simulink model "truck_fra_oven_konstant_hastighet"  (R2019b)
settings: Solver=VariableStepAuto  StartTime=0.0  StopTime=10.0  MaxStep=0.01  RelTol=1e-3
settings Model: EnablePacing=on  Creator=hansae  LastModifiedBy=hansae
settings DebuggingCC: UnconnectedInputMsg=none  UnconnectedOutputMsg=none  UnconnectedLineMsg=none  SFMachineParentedDataDiag=error
settings ModelReferenceCC: EnableRefExpFcnMdlSchedulingChecks=off
settings RTWCC: Description=Generic Real-Time Target

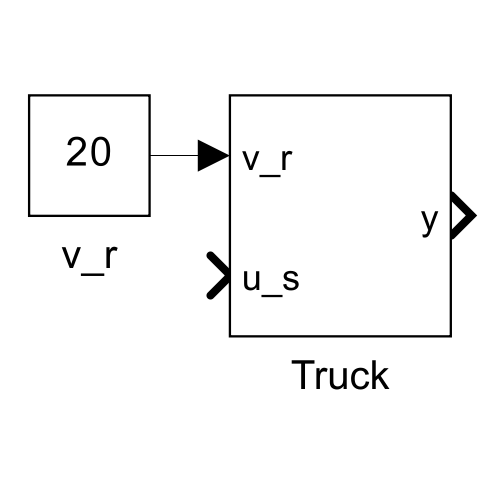
[thumbnail: Simulink's stored preview of the top-level diagram]
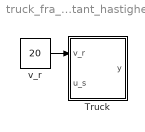
== system truck_fra_oven_konstant_hastighet ==
  Truck : Subsystem
  v_r : Constant  Value=20
  wires:
  v_r/1 -> Truck/1(v_r)

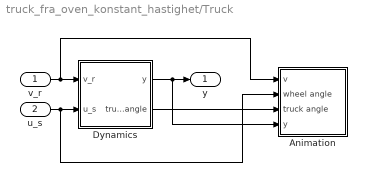
== system truck_fra_oven_konstant_hastighet/Truck ==
  v_r : Inport
  u_s : Inport  Port=2
  Animation : Subsystem
  Dynamics : Subsystem  ClipboardFcn=parameters_truck.m
  y : Outport
  wires:
  Dynamics/1(y) -> Animation/4(y), y/1
  u_s/1 -> Animation/2(wheel angle), Dynamics/2(u_s)
  v_r/1 -> Animation/1(v), Dynamics/1(v_r)
  Dynamics/2(truck angle) -> Animation/3(truck angle)

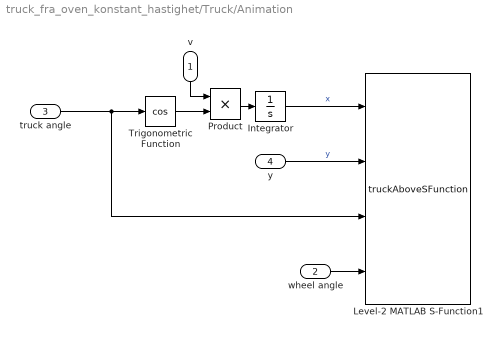
== system truck_fra_oven_konstant_hastighet/Truck/Animation ==
  v : Inport
  wheel angle : Inport  Port=2
  truck angle : Inport  Port=3
  y : Inport  Port=4
  Integrator : Integrator
  Level-2 MATLAB S-Function1 : M-S-Function  FunctionName=truckAboveSFunction
  Product : Product
  Trigonometric Function : Trigonometry  Operator=cos
  wires:
  Product/1 -> Integrator/1
  Trigonometric Function/1 -> Product/2
  v/1 -> Product/1
  y/1 -> Level-2 MATLAB S-Function1/2  "y"
  Integrator/1 -> Level-2 MATLAB S-Function1/1  "x"
  truck angle/1 -> Trigonometric Function/1, Level-2 MATLAB S-Function1/3
  wheel angle/1 -> Level-2 MATLAB S-Function1/4

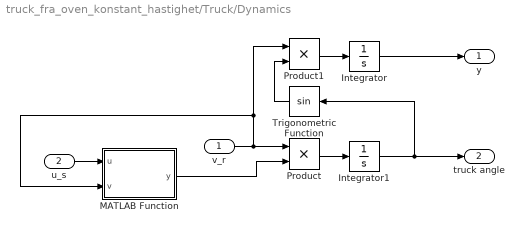
== system truck_fra_oven_konstant_hastighet/Truck/Dynamics ==
  v_r : Inport
  u_s : Inport  Port=2
  Integrator : Integrator  InitialCondition=-2
  Integrator1 : Integrator
  MATLAB Function : MATLAB Function  TreatAsAtomicUnit=on
  Product : Product
  Product1 : Product
  Trigonometric Function : Trigonometry
  y : Outport
  truck angle : Outport  Port=2
  wires:
  Integrator/1 -> y/1
  Integrator1/1 -> truck angle/1, Trigonometric Function/1
  Product/1 -> Integrator1/1
  v_r/1 -> MATLAB Function/2(v), Product1/1, Product/1
  Product1/1 -> Integrator/1
  Trigonometric Function/1 -> Product1/2
  u_s/1 -> MATLAB Function/1(u)
  MATLAB Function/1(y) -> Product/2

== matlab function truck_fra_oven_konstant_hastighet/Truck/Dynamics/MATLAB Function ==
  data: u input; y output; v input
function y = saturation(u,v)
    Pmax = 400000;
    epsilon = 0.1;
    
    sat = Pmax/sqrt(v^2+epsilon);
    y = max(min(u,sat),-sat);
